simulink model "load_test"  (R2021a)
settings: Solver=VariableStepAuto  StartTime=0.0  StopTime=200  MaxStep=1e-4  RelTol=1e-3
libraries: spsRMSLib x8, spsVoltageMeasurementLib x4, spsCurrentMeasurementLib x3, spsBreakerLib x2, spsAsynchronousMachinepuUnitsLib x1, spsDCMachineLib x1, spsPower3phInstantaneousLib x1, spsSeriesRLCBranchLib x1, simulink x1, nesl_utility x1, spsThreePhaseVIMeasurementLib x1, spsThreePhaseBreakerLib x1
settings Model: Creator=DELL  LastModifiedBy=HP
settings SolverCC: ZeroCrossAlgorithm=Adaptive  AlgebraicLoopSolver=TrustRegion
settings DataIOCC: ReturnWorkspaceOutputs=off
settings DebuggingCC: IgnoredZcDiagnostic=none  PregeneratedLibrarySubsystemCodeDiagnostic=none  SFMachineParentedDataDiag=warning  ArithmeticOperatorsInVariantConditions=warning
settings SFSimCC: SimUseLocalCustomCode=off  CustomCodeUndefinedFunction=UseInterfaceOnly
settings RTWCC: RTWUseLocalCustomCode=off

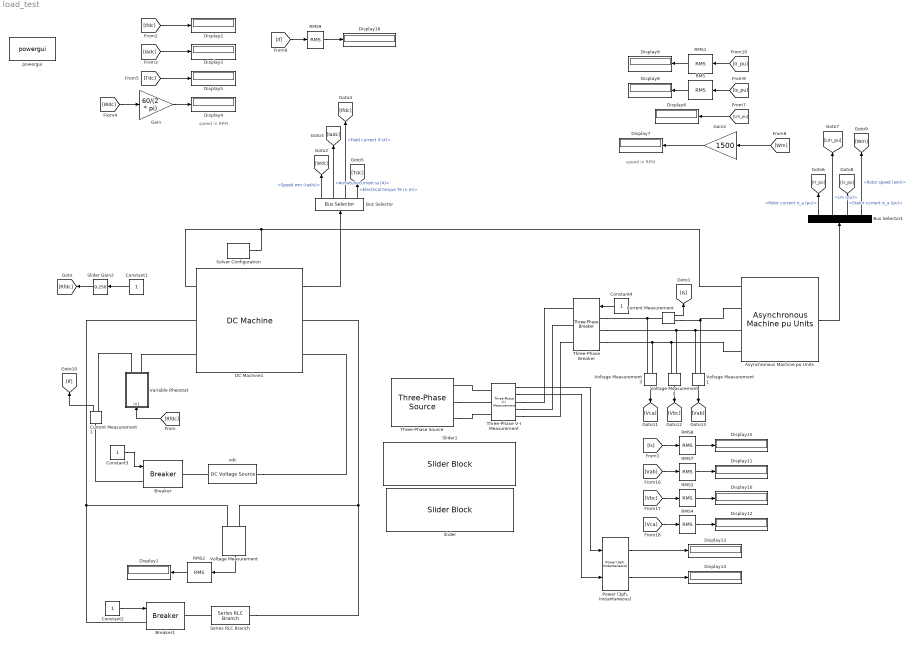
== system load_test ==
  note: speed in RPM
  note: speed in RPM
  Asynchronous Machine pu Units : spsAsynchronousMachinepuUnitsLib/Asynchronous Machine pu Units  RotorType=Squirrel-cage  PresetModel=No  MechanicalLoad=Mechanical rotational port  ShowDetailedParameters=on  ReferenceFrame=Rotor  Units=pu  MeasurementBus=off  NominalParameters=[1.5e+04 400 50]  VoltageRatio=1  Stator=[0.02013 0.02919]  Rotor=[0.02067 0.02919]  Cage1=[0.01909 0.0397]  Cage2=[0.01909 0.0397]  Lm=1.89  Mechanical=[0.1 0.05 2]  PolePairs=2  InitialConditions="[ 1,0   0,0,0   0,0,0 ]"  SimulateSaturation=off  Saturation="[0.212,0.4201,0.8125,1.0979,1.4799,2.2457,3.2586,4.5763,6.4763 ;   0.5,0.7,0.9,1,1.1,1.2 ,1.3,1.4,1.5]"  LoadFlowParameters=0  TsPowergui=0  TsBlock=-1  IterativeModel=Trapezoidal non iterative  IterativeDiscreteModel=Trapezoidal non iterative  Pmec=0
      settings: SourceProductBaseCode=PS
  Breaker : spsBreakerLib/Breaker  InitialState=0  SwitchingTimes="[1/60  5/60]"  External=on  BreakerResistance=0.01  SnubberResistance=1e6  SnubberCapacitance=inf  Measurements=None  MoreParameters=on  NoBreakLoop=off
      settings: SourceProductBaseCode=PS
  Breaker1 : spsBreakerLib/Breaker  InitialState=0  SwitchingTimes="[1/60  5/60]"  External=on  BreakerResistance=0.01  SnubberResistance=1e6  SnubberCapacitance=inf  Measurements=None  MoreParameters=on  NoBreakLoop=off
      settings: SourceProductBaseCode=PS
  Bus Selector : BusSelector  OutputSignals=Speed wm (rad/s),Armature current ia (A),Field current if (A),Electrical torque Te (n m)
  Bus Selector1 : BusSelector  OutputSignals=Rotor measurements.Rotor current ir_a (pu),Lm (pu),Stator measurements.Stator current is_a (pu),Mechanical.Rotor speed (wm)
  Constant{1..4} (4 alike) : Constant
  Current Measurement : spsCurrentMeasurementLib/Current Measurement  PhasorSimulation=off  OutputType=Complex  PSBequivalent=0
  Current Measurement1 : spsCurrentMeasurementLib/Current Measurement  PhasorSimulation=off  OutputType=Complex  PSBequivalent=0
  DC Machine1 : spsDCMachineLib/DC Machine  PresetModel=No  MechanicalLoad=Mechanical rotational port  FieldType=Wound  ShowDetailedParameters=on  MeasurementBus=off  RLa=[0.9875 0.01244]  RLf=[130.1 20.82]  Laf=0.8355  MachineConstant=Torque constant (N.m/A)  Ke=1.8  Kt=1.8  J=0.1239  Bm=0.15  Tf=3.164  w0=0  Ifinit=0.000349954470923333  TsPowergui=0  TsBlock=-1
  Display{1..16} (16 alike) : Display
  Gain : Gain  Gain=60/(2 * pi)
  Gain2 : Gain  Gain=1500
  "Power (3ph, Instantaneous)" : spsPower3phInstantaneousLib/Power (3ph, Instantaneous)
  RMS{,1..4,7..9} (8 alike) : spsRMSLib/RMS  TrueRMS=on  Freq=50  RMSInit=0  Ts=0
  Series RLC Branch : spsSeriesRLCBranchLib/Series RLC Branch  LConnTagsString=__new0  RConnTagsString=__new0  BranchType=R  Resistance=50  Inductance=1e-3  SetiL0=off  InitialCurrent=0  Capacitance=1e-6  Setx0=off  InitialVoltage=0  Measurements=None
  Slider : SliderBlock  ScaleMax=400
  Slider Gain2 : simulink/Math Operations/Slider Gain  gain=0.250  low=0  high=25
  Slider1 : SliderBlock  ScaleMax=50
  Solver Configuration : nesl_utility/Solver Configuration  PhysicalDomain=network_engine_domain  SubClassName=solver  LeftPortType=input  RightPortType=generic  Tones=[]  Harmonics=[]  SimulateNoise=off  Profile=off  UseLocalSampling=off  EnableSwitchedLinearOptims=on  FrequencyDomain=off  UseCCode=off  RelTol=0.001  AbsTol=1e-06  MinStep=1e-09  ToWorkspace=off  RevertToSquareIcSolve=off  NumHomotopyIterations=100  PhasorMode=off  PhasorModeNumHarmonics=1  DoDC=off  ResidualTolerance=1e-09  UseLocalSolver=off  LocalSolverChoice=NE_BACKWARD_EULER_ADVANCER  LocalSolverSampleTime=0.001  DoFixedCost=off  MaxNonlinIter=3  MaxModeIter=2  ComputeImpulses=off  ImpulseIterations=2  LinearAlgebra=Sparse  EquationFormulation=NE_TIME_EF  DelaysMemoryBudget=1024  AutomaticFiltering=on  FilteringTimeConstant=0.001  PartitionStorageMethod=AS_NEEDED  PartitionMemoryBudget=1024  PartitionMethod=FAST
      settings: SourceProductBaseCode=PW,SS
  Three-Phase V-I Measurement : spsThreePhaseVIMeasurementLib/Three-Phase V-I Measurement  VoltageMeasurement=phase-to-ground  SetLabelV=off  LabelV=Vabc  Vpu=off  VpuLL=off  CurrentMeasurement=yes  SetLabelI=off  LabelI=Iabc  Ipu=off  Pbase=100e6  Vbase=500e3  OutputType=Complex  PhasorSimulation=off  PSBequivalent=0
  Three-Phase Breaker : spsThreePhaseBreakerLib/Three-Phase Breaker  InitialState=open  SwitchA=on  SwitchB=on  SwitchC=on  SwitchTimes=[0.1]  External=on  BreakerResistance=0.001  SnubberResistance=1e6  SnubberCapacitance=inf  Measurements=None
  Three-Phase Source : spsThreePhaseSourceLib/Three-Phase Source  InternalConnection=Yg  VoltagePhases=off  Voltage=400  PhaseAngle=0  Voltage_phases=[25e3 25e3 25e3]/sqrt(3)  PhaseAngles_phases=[0 -120 +120]  Frequency=50  NonIdealSource=off  SpecifyImpedance=off  Resistance=0.8929  Inductance=16.58e-3  ShortCircuitLevel=100e6  BaseVoltage=25e3  XRratio=7  BusType=swing  Pref=10e3  Qref=0  Prefabc=[10e3, 10e3, 10e3]  Qrefabc=[0, 0, 0]  Qmin=-inf  Qmax=inf
  Variable Rheostat : Subsystem
  Voltage Measurement{,1..3} (4 alike) : spsVoltageMeasurementLib/Voltage Measurement  PhasorSimulation=off  OutputType=Complex  PSBequivalent=0
  powergui : spspowerguiLib/powergui  Priority=1  SimulationMode=Continuous  SampleTime=1e-6  frequency=50  Iterations=50  frequencyindice=0  Pbase=100e6  ErrMax=1e-4  UnitsV=kV  UnitsW=MW  buscounter=0  FunctionMessages=off  echomessages=off  EnableUseOfTLC=off  CurrentSourceSwitches=off  DisableSnubberDevices=off  DisableRonSwitches=off  DisableVfSwitches=off  DisplayEquations=off  AutomaticDiscreteSolvers=off  SolverType=Tustin/Backward Euler (TBE)  Interpol=off  ExternalGateDelay=off  methode=off  Ts=100  x0status=blocks  SPID=on  SwTol=0  HookPort=off  NonlinearTolerance=1e-4  nMaxIteration=100  ContinueOnMaxIteration=off  RestoreLinks=warning  ResistiveCurrentMeasurement=off  Frange=[0:2:500]  Ylog=off  Xlog=on  ShowGrid=off  save=off  variable=ZData  structure=0  ZoomFFT=off  StartTime=0.0  cycles=1  DisplayStyle=1  fundamental=60  FreqAxis=off  MaxFrequency=1000  frequencyindicesteady=1  RmsSteady=1  display=off
  "vdc " : spsDCVoltageSourceLib/DC Voltage Source  Amplitude=350  Measurements=None
  wires:
  [Rfdc] -> Variable Rheostat/1(In1)
  Constant1/1 -> Slider Gain2/1
  Slider Gain2/1 -> [Rfdc]
  DC Machine1/1 -> Bus Selector/1
  Bus Selector/1 -> [Wdc]  "<Speed wm (rad/s)>"
  Bus Selector/2 -> [Iadc]  "<Armature current ia (A)>"
  Bus Selector/3 -> [Ifdc]  "<Field current if (A)>"
  Bus Selector/4 -> [Tdc]  "<Electrical torque Te (n m)>"
  [Tdc] -> Display5/1
  [Wdc] -> Gain/1
  [Ifdc] -> Display2/1
  [Iadc] -> Display3/1
  Gain/1 -> Display4/1
  Constant4/1 -> Three-Phase Breaker/1
  Asynchronous Machine pu Units/1 -> Bus Selector1/1
  Constant3/1 -> Breaker/1
  Bus Selector1/1 -> [Ir_pu]  "<Rotor current ir_a (pu)>"
  Bus Selector1/2 -> [Lm_pu]  "<Lm (pu)>"
  Bus Selector1/3 -> [Is_pu]  "<Stator current is_a (pu)>"
  Bus Selector1/4 -> [Wm]  "<Rotor speed (wm)>"
  Gain2/1 -> Display7/1
  [Is_pu] -> RMS/1
  [Ir_pu] -> RMS1/1
  [Wm] -> Gain2/1
  RMS1/1 -> Display9/1
  RMS/1 -> Display8/1
  [Lm_pu] -> Display6/1
  RMS2/1 -> Display1/1
  Voltage Measurement/1 -> RMS2/1
  Constant2/1 -> Breaker1/1
  Voltage Measurement1/1 -> [Vab]
  Voltage Measurement3/1 -> [Vca]
  Voltage Measurement2/1 -> [Vbc]
  [Vab] -> RMS7/1
  RMS7/1 -> Display11/1
  RMS3/1 -> Display10/1
  [Vbc] -> RMS3/1
  RMS4/1 -> Display12/1
  [Vca] -> RMS4/1
  Three-Phase V-I Measurement/1 -> "Power (3ph, Instantaneous)"/1
  Three-Phase V-I Measurement/2 -> "Power (3ph, Instantaneous)"/2
  "Power (3ph, Instantaneous)"/1 -> Display13/1
  "Power (3ph, Instantaneous)"/2 -> Display14/1
  Current Measurement/1 -> [Is]
  RMS8/1 -> Display15/1
  [Is] -> RMS8/1
  Current Measurement1/1 -> [If]
  RMS9/1 -> Display16/1
  [If] -> RMS9/1
  connections:
  DC Machine1/LConn1 -- Solver Configuration/RConn1 -- Asynchronous Machine pu Units/LConn1
  Variable Rheostat/RConn2 -- DC Machine1/LConn3
  Breaker/LConn1 -- Current Measurement1/LConn1
  "vdc "/LConn1 -- DC Machine1/RConn2
  Three-Phase Breaker/LConn1 -- Voltage Measurement3/LConn2 -- Current Measurement/LConn1
  Three-Phase Breaker/LConn2 -- Voltage Measurement2/LConn1 -- Voltage Measurement1/LConn2 -- Asynchronous Machine pu Units/LConn3
  Three-Phase Breaker/LConn3 -- Voltage Measurement3/LConn1 -- Voltage Measurement2/LConn2 -- Asynchronous Machine pu Units/LConn4
  Three-Phase V-I Measurement/LConn1 -- Three-Phase Source/RConn1
  Three-Phase Source/RConn2 -- Three-Phase V-I Measurement/LConn2
  Three-Phase Source/RConn3 -- Three-Phase V-I Measurement/LConn3
  "vdc "/RConn1 -- Breaker/RConn1
  Voltage Measurement/LConn2 -- Series RLC Branch/RConn1 -- DC Machine1/RConn1
  Voltage Measurement/LConn1 -- Breaker1/LConn1 -- DC Machine1/LConn2
  Series RLC Branch/LConn1 -- Breaker1/RConn1
  Three-Phase V-I Measurement/RConn1 -- Three-Phase Breaker/RConn1
  Three-Phase V-I Measurement/RConn2 -- Three-Phase Breaker/RConn2
  Three-Phase V-I Measurement/RConn3 -- Three-Phase Breaker/RConn3
  Current Measurement/RConn1 -- Asynchronous Machine pu Units/LConn2 -- Voltage Measurement1/LConn1
  Current Measurement1/RConn1 -- Variable Rheostat/RConn1

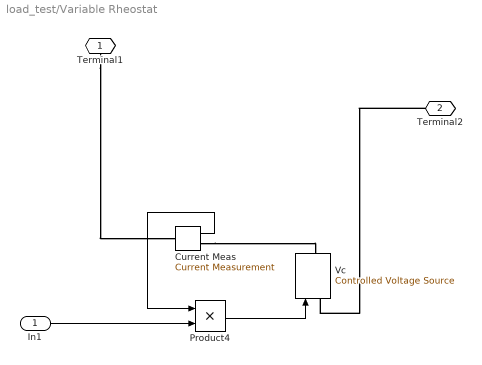
== system load_test/Variable Rheostat ==
  In1 : Inport
  Current Meas : spsCurrentMeasurementLib/Current Measurement  PhasorSimulation=off  OutputType=Complex  PSBequivalent=0
  Product4 : Product
  Vc : spsControlledVoltageSourceLib/Controlled Voltage Source  Initialize=on  Source_Type=DC  Amplitude=0  Phase=0  Frequency=0  Measurements=None
  Terminal1 : PMIOPort  Side=Right
  Terminal2 : PMIOPort  Port=2  Side=Right
  wires:
  Current Meas/1 -> Product4/1
  In1/1 -> Product4/2
  Product4/1 -> Vc/1
  connections:
  Terminal2/RConn1 -- Vc/LConn1
  Terminal1/RConn1 -- Current Meas/LConn1
  Current Meas/RConn1 -- Vc/RConn1
